simulink model "second_control"  (R2021b)
settings: Solver=VariableStepAuto  StartTime=0.0  StopTime=0.01  RelTol=1e-3
undefined symbols (not defined in the file): Ion, Lithium
libraries: spsMosfetLib x8, spsSeriesRLCBranchLib x6, eeDcVoltageController x4, spsVoltageMeasurementLib x4, spsCurrentMeasurementLib x3, eeDcCurrentController x3, spsACVoltageSourceLib x1, spsBatteryLib x1, spsPLLLib x1, simulink x1, spspowerguiLib x1
settings Model: Creator=eee  LastModifiedBy=eee

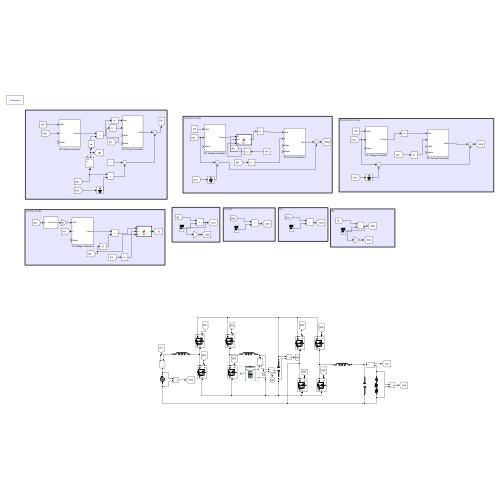
[thumbnail: Simulink's stored preview of the top-level diagram]
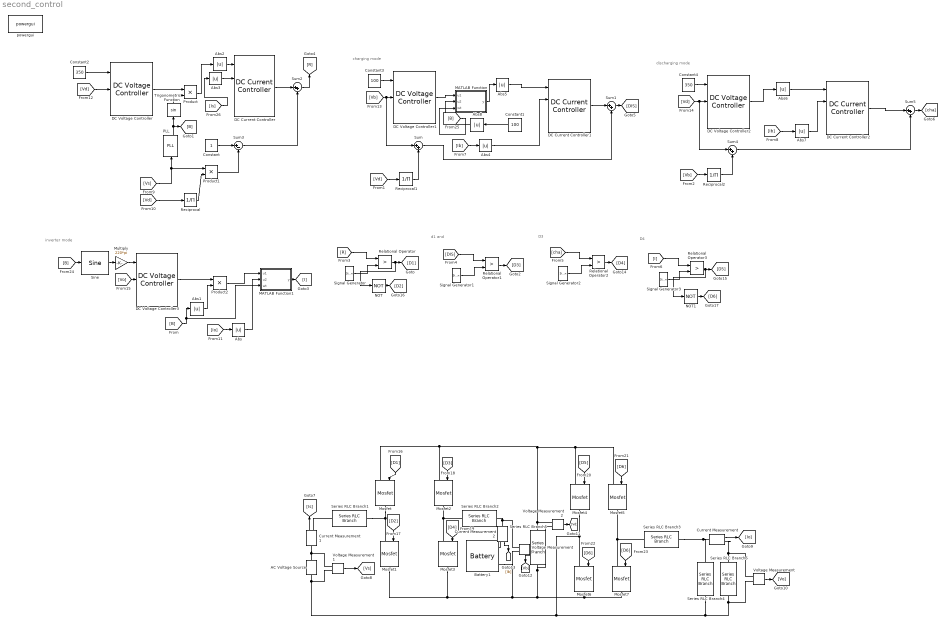
== system second_control ==
  note: D4
  note: D3
  note: d1 and
  note: inverter mode
  note: charging mode
  note: discharging mode
  AC Voltage Source : spsACVoltageSourceLib/AC Voltage Source  Amplitude=220*pi  Phase=0  Frequency=60  SampleTime=0  Measurements=None  BusType=swing  Pref=10e3  Qref=0  Qmin=-inf  Qmax=+inf
  Abs{,1..8} (9 alike) : Abs
  Battery1 : spsBatteryLib/Battery  BatType=Lithium-Ion  ShowTempParam=off  ThermalPreset=no  ShowAgeParam=off  NomV=192  NomQ=100  SOC=100  Batt_Tr=30  PresetModel=on  MaxQ=100  MinV=144  FullV=223.4855  Dis_rate=43.4783  R=0.0192  Normal_OP=90.4348  expZone="[207.4341      4.913043]"  current=[6.5 13 32.5]  Units=Time  Tci=20  NomT=20  T2=-30  MaxQ2=4.8  FullV2=7.1  Normal_OP2=5.655  expZone2="[6.58           1]"  Rca=0.6  ti=2000  Dp=0  Neq0=0  Tsim=1e6  Ta1=25  Qeol=5.4*0.9  Reol=0.013333*1.2  Char_age=[2.3478, 3]  Dis_age=[2.3478, 10]  N1=1500  N2=10500  N3=1000  N4=1400  Ta2=45  N5=950
  Constant : Constant
  Constant1 : Constant  Value=100
  Constant2 : Constant  Value=350
  Constant3 : Constant  Value=100
  Constant4 : Constant  Value=350
  Current Measurement : spsCurrentMeasurementLib/Current Measurement  PhasorSimulation=off  OutputType=Complex  PSBequivalent=0
  Current Measurement1 : spsCurrentMeasurementLib/Current Measurement  PhasorSimulation=off  OutputType=Complex  PSBequivalent=0
  Current Measurement2 : spsCurrentMeasurementLib/Current Measurement  PhasorSimulation=off  OutputType=Complex  PSBequivalent=0
  DC Current Controller : eeDcCurrentController/DC Current Controller  Kp=1  Ki=5  Kaw=1  VoltLim=Positive voltage only  Ts=-1  Tsd=0.001  ActZC=off
      settings: SourceProductBaseCode=PS
  DC Current Controller1 : eeDcCurrentController/DC Current Controller  Kp=1  Ki=5  Kaw=1  VoltLim=Positive and negative voltage  Ts=-1  Tsd=0.001  ActZC=off
      settings: SourceProductBaseCode=PS
  DC Current Controller2 : eeDcCurrentController/DC Current Controller  Kp=1  Ki=5  Kaw=1  VoltLim=Positive and negative voltage  Ts=-1  Tsd=0.001  ActZC=off
      settings: SourceProductBaseCode=PS
  DC Voltage Controller{,1..3} (4 alike) : eeDcVoltageController/DC Voltage Controller  Kp=0.1  Ki=50  Kaw=1  up=1  lo=0  Ts=-1  Tsd=0.001  Tf=0.001  ActZC=off  ActVdcFilter=on
      settings: SourceProductBaseCode=PS
  MATLAB Function : MATLAB Function  TreatAsAtomicUnit=on
  MATLAB Function1 : MATLAB Function  TreatAsAtomicUnit=on
  Mosfet{,1..7} (8 alike) : spsMosfetLib/Mosfet  Ron=0.1  Lon=0  Rd=0.01  Vfd=0  IC=0  Rs=1e5  Cs=inf  Measurements=off
  Multiply : Gain  Gain=220*pi
  NOT : Logic  Operator=NOT  IconShape=distinctive  AllPortsSameDT=off  OutDataTypeStr=boolean
  NOT1 : Logic  Operator=NOT  IconShape=distinctive  AllPortsSameDT=off  OutDataTypeStr=boolean
  PLL : spsPLLLib/PLL  Fmin=45  Par_Init=[0, 60]  ParK=[180, 3200, 1]  TcD=1e-4  MaxRateChangeFreq=12  FilterCutOffFreq=25  Ts=0  AGC=on
      settings: SourceProductBaseCode=PS
  Product : Product
  Product1 : Product
  Product2 : Product
  Reciprocal : Product  Inputs=/
  Reciprocal1 : Product  Inputs=/
  Reciprocal2 : Product  Inputs=/
  Relational Operator{,1..3} (4 alike) : RelationalOperator  Operator=>  OutDataTypeStr=boolean  RndMeth=Simplest
  Series RLC Branch1 : spsSeriesRLCBranchLib/Series RLC Branch  LConnTagsString=__new0  RConnTagsString=__new0  BranchType=L  Resistance=1  Inductance=1.5*1e-3  SetiL0=off  InitialCurrent=0  Capacitance=1e-6  Setx0=off  InitialVoltage=0  Measurements=None
  Series RLC Branch2 : spsSeriesRLCBranchLib/Series RLC Branch  LConnTagsString=__new0  RConnTagsString=__new0  BranchType=L  Resistance=1  Inductance=1.5*1e-3  SetiL0=off  InitialCurrent=0  Capacitance=1e-6  Setx0=off  InitialVoltage=0  Measurements=None
  Series RLC Branch3 : spsSeriesRLCBranchLib/Series RLC Branch  LConnTagsString=__new0  RConnTagsString=__new0  BranchType=L  Resistance=1  Inductance=1.5*1e-3  SetiL0=off  InitialCurrent=0  Capacitance=1e-6  Setx0=off  InitialVoltage=0  Measurements=None
  Series RLC Branch4 : spsSeriesRLCBranchLib/Series RLC Branch  LConnTagsString=__new0  RConnTagsString=__new0  BranchType=C  Resistance=1  Inductance=1e-3  SetiL0=off  InitialCurrent=0  Capacitance=30*1e-6  Setx0=off  InitialVoltage=0  Measurements=None
  Series RLC Branch5 : spsSeriesRLCBranchLib/Series RLC Branch  LConnTagsString=__new0  RConnTagsString=__new0  BranchType=C  Resistance=1  Inductance=1e-3  SetiL0=off  InitialCurrent=0  Capacitance=2*680*1e-6  Setx0=off  InitialVoltage=0  Measurements=None
  Series RLC Branch6 : spsSeriesRLCBranchLib/Series RLC Branch  LConnTagsString=__new0  RConnTagsString=__new0  BranchType=RLC  Resistance=1  Inductance=1e-3  SetiL0=off  InitialCurrent=0  Capacitance=1e-6  Setx0=off  InitialVoltage=0  Measurements=None
  Signal Generator{,1..3} (4 alike) : SignalGenerator  WaveForm=sawtooth  Frequency=20000
  Sine : simulink/Lookup Tables/Sine  Formula=sin(2*pi*u)  NumDataPoints=(2^5)+1  OutputWordLength=16  InternalRulePriority=Speed
  Sum{,1..2,4..5} (5 alike) : Sum  Inputs=|++
  Sum3 : Sum  Inputs=|+-
  Trigonometric Function : Trigonometry
  Voltage Measurement{,1..3} (4 alike) : spsVoltageMeasurementLib/Voltage Measurement  PhasorSimulation=off  OutputType=Complex  PSBequivalent=0
  powergui : spspowerguiLib/powergui  Priority=1  SimulationMode=Continuous  SampleTime=50e-6  frequency=60  Iterations=50  frequencyindice=60  Pbase=100e6  ErrMax=1e-4  UnitsV=kV  UnitsW=MW  buscounter=0  FunctionMessages=off  echomessages=off  EnableUseOfTLC=off  CurrentSourceSwitches=off  DisableSnubberDevices=off  DisableRonSwitches=off  DisableVfSwitches=off  DisplayEquations=off  AutomaticDiscreteSolvers=off  SolverType=Tustin/Backward Euler (TBE)  Interpol=off  ExternalGateDelay=off  methode=off  Ts=100  x0status=blocks  SPID=on  SwTol=0  HookPort=off  NonlinearTolerance=1e-4  nMaxIteration=100  ContinueOnMaxIteration=off  RestoreLinks=warning  ResistiveCurrentMeasurement=off  Frange=[0:2:500]  Ylog=off  Xlog=on  ShowGrid=off  save=off  variable=ZData  structure=0  ZoomFFT=off  StartTime=0.0  cycles=1  DisplayStyle=1  fundamental=60  FreqAxis=off  MaxFrequency=1000  frequencyindicesteady=1  RmsSteady=1  display=off
  wires:
  Sum3/1 -> Sum2/2
  Trigonometric Function/1 -> Product/2
  [Vd] -> Reciprocal/1
  Reciprocal/1 -> Product1/2
  Constant/1 -> Sum3/1
  DC Voltage Controller/1 -> Product/1
  Constant2/1 -> DC Voltage Controller/1
  [Vd] -> DC Voltage Controller/2
  [Vs] -> Product1/1, PLL/1
  PLL/2 -> [B], Trigonometric Function/1
  DC Current Controller/1 -> Sum2/1
  Product1/1 -> Sum3/2
  Sum2/1 -> [R]
  [Vb] -> Sum/1, DC Voltage Controller1/2
  Constant3/1 -> DC Voltage Controller1/1
  DC Voltage Controller1/1 -> MATLAB Function/1(u1)
  [Vd] -> Reciprocal1/1
  Reciprocal1/1 -> Sum/2
  DC Current Controller1/1 -> Sum1/1
  Sum/1 -> Sum1/2
  Constant4/1 -> DC Voltage Controller2/1
  Reciprocal2/1 -> Sum4/2
  [Vb] -> Reciprocal2/1
  DC Current Controller2/1 -> Sum5/1
  [Vd] -> Sum4/1, DC Voltage Controller2/2
  Sum4/1 -> Sum5/2
  DC Voltage Controller3/1 -> Product2/1
  Product2/1 -> MATLAB Function1/1(u1)
  [Io] -> Abs/1
  Abs/1 -> MATLAB Function1/2(u2)
  [B] -> MATLAB Function1/3(wt), Abs1/1
  Abs1/1 -> Product2/2
  Abs2/1 -> DC Current Controller/1
  Product/1 -> Abs2/1
  Abs3/1 -> DC Current Controller/2
  [Is] -> Abs3/1
  [Ib] -> Abs4/1
  MATLAB Function/1(y) -> Abs5/1
  Abs5/1 -> DC Current Controller1/1
  DC Voltage Controller2/1 -> Abs6/1
  Abs6/1 -> DC Current Controller2/1
  [Ib] -> Abs7/1
  Abs7/1 -> DC Current Controller2/2
  Abs4/1 -> DC Current Controller1/2
  Constant1/1 -> Abs8/1
  Signal Generator/1 -> Relational Operator/2
  [R] -> Relational Operator/1
  MATLAB Function1/1(y) -> [I]
  Sum1/1 -> [DIS]
  Sum5/1 -> [cha]
  [DIS] -> Relational Operator1/1
  Signal Generator1/1 -> Relational Operator1/2
  Relational Operator1/1 -> [D3]
  [cha] -> Relational Operator2/1
  Signal Generator2/1 -> Relational Operator2/2
  Relational Operator2/1 -> [D4]
  Signal Generator3/1 -> Relational Operator3/2
  Relational Operator3/1 -> NOT1/1, [D5]
  [I] -> Relational Operator3/1
  Current Measurement1/1 -> [Is]
  Voltage Measurement1/1 -> [Vs]
  Current Measurement/1 -> [Io]
  Voltage Measurement/1 -> [Vo]
  Voltage Measurement2/1 -> [Vd]
  Voltage Measurement3/1 -> [Vb]
  Current Measurement2/1 -> [Ib]
  [Vo] -> DC Voltage Controller3/2
  Relational Operator/1 -> NOT/1, [D1]
  NOT/1 -> [D2]
  NOT1/1 -> [D6]
  [D1] -> Mosfet/1
  [D2] -> Mosfet1/1
  [D3] -> Mosfet2/1
  [D4] -> Mosfet3/1
  [D5] -> Mosfet4/1
  [D6] -> Mosfet5/1
  [D6] -> Mosfet6/1
  [D6] -> Mosfet7/1
  [B] -> Sine/1
  Sine/1 -> Multiply/1
  Multiply/1 -> DC Voltage Controller3/1
  Abs8/1 -> MATLAB Function/2(u2)
  [B] -> MATLAB Function/3(wt)
  connections:
  Mosfet/RConn1 -- Mosfet1/LConn1 -- Series RLC Branch1/LConn1
  Mosfet3/LConn1 -- Series RLC Branch2/RConn1 -- Mosfet2/RConn1
  Mosfet1/RConn1 -- Mosfet3/RConn1 -- Voltage Measurement3/LConn2 -- Battery1/LConn2 -- Voltage Measurement2/LConn2 -- Series RLC Branch5/LConn1 -- Mosfet6/RConn1 -- Mosfet7/RConn1
  AC Voltage Source/LConn1 -- Voltage Measurement1/LConn2 -- Mosfet6/LConn1 -- Mosfet4/RConn1 -- Series RLC Branch4/LConn1 -- Voltage Measurement/LConn2 -- Series RLC Branch6/LConn1
  Mosfet/LConn1 -- Voltage Measurement2/LConn1 -- Series RLC Branch5/RConn1 -- Mosfet5/LConn1 -- Mosfet4/LConn1 -- Mosfet2/LConn1
  Mosfet7/LConn1 -- Series RLC Branch3/RConn1 -- Mosfet5/RConn1
  Series RLC Branch3/LConn1 -- Series RLC Branch4/RConn1 -- Current Measurement/LConn1
  Current Measurement/RConn1 -- Voltage Measurement/LConn1 -- Series RLC Branch6/RConn1
  Current Measurement1/LConn1 -- Voltage Measurement1/LConn1 -- AC Voltage Source/RConn1
  Current Measurement1/RConn1 -- Series RLC Branch1/RConn1
  Series RLC Branch2/LConn1 -- Voltage Measurement3/LConn1 -- Current Measurement2/LConn1
  Current Measurement2/RConn1 -- Battery1/LConn1

== matlab function second_control/MATLAB Function ==
  data: u1 input; y output; u2 input; wt input
function y = fcn(u1,u2,wt)
Io=u2;
d=u1;
OC=1.1*Io;
CL=1.2*OC;
sin_ref=sin(wt);
if Io>=OC
    
        sin_limit=0;
        mode=current_limit;
    
else
    
        if Io>=cl
        
            sin_limit=sin_ref;
            mode=current_limit;
        end
end
    
if (mode==current_limit)
    
        if(sin(wt>0)&&sin_limit<=sin_ref)
        
            sin_ref=sin_limit+(kp*(CL-abs(Io)));
        
        else
            
                if(sin(wt<0&&sin_limit>=sin_ref))
                
                    sin_ref=sin_limit-(kp*(CL-abs(Io)));
                
                else
                
                    mode=normal;
                end
        end
end
if(mode==normal)

else
    d=m*sin_ref;
end
y = d;

== matlab function second_control/MATLAB Function1 ==
  data: u1 input; y output; u2 input; wt input
function y = fcn(u1,u2,wt)
Io=u2;
d=u1;
OC=1.1*Io;
CL=1.2*OC;
sin_ref=sin(wt);
if Io>=OC
    
        sin_limit=0;
        mode=current_limit;
    
else
    
        if Io>=cl
        
            sin_limit=sin_ref;
            mode=current_limit;
        end
end
    
if (mode==current_limit)
    
        if(sin(wt)>0&&sin_limit<=sin_ref)
        
            sin_ref=sin_limit+(kp*(CL-abs(Io)));
        
        else
            
                if(sin(wt<0&&sin_limit>=sin_ref))
                
                    sin_ref=sin_limit-(kp*(CL-abs(Io)));
                
                else
                
                    mode=normal;
                end
        end
end
if(mode==normal)

else
    d=m*sin_ref;
end
y = d;
